simulink model "FinalTest_21_3"  (R2022b)
settings: Solver=FixedStepAuto  StartTime=0.0  StopTime=20  FixedStep=0.001  MaxStep=0.001  RelTol=1e-3
undefined symbols (not defined in the file): h, km, m, s, sigbuilder_block, smiData, X, Y, Z
libraries: sm_lib x105, aerolibconvert2 x14, nesl_utility x6, simulink_extras x4, vehdynlibsteering x1, autolibshared x1
(part 1 of 3)
settings Model: Creator=Lenovo  LastModifiedBy=Lenovo

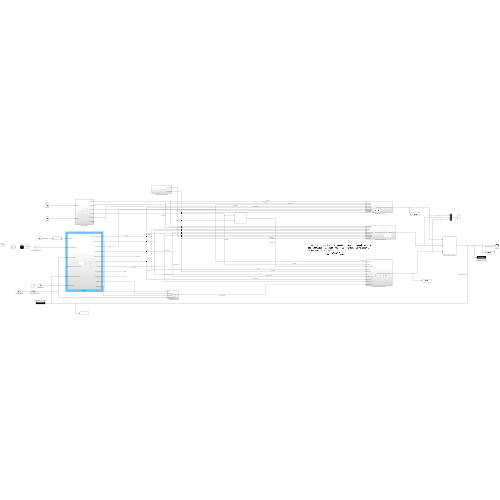
[thumbnail: Simulink's stored preview of the top-level diagram]
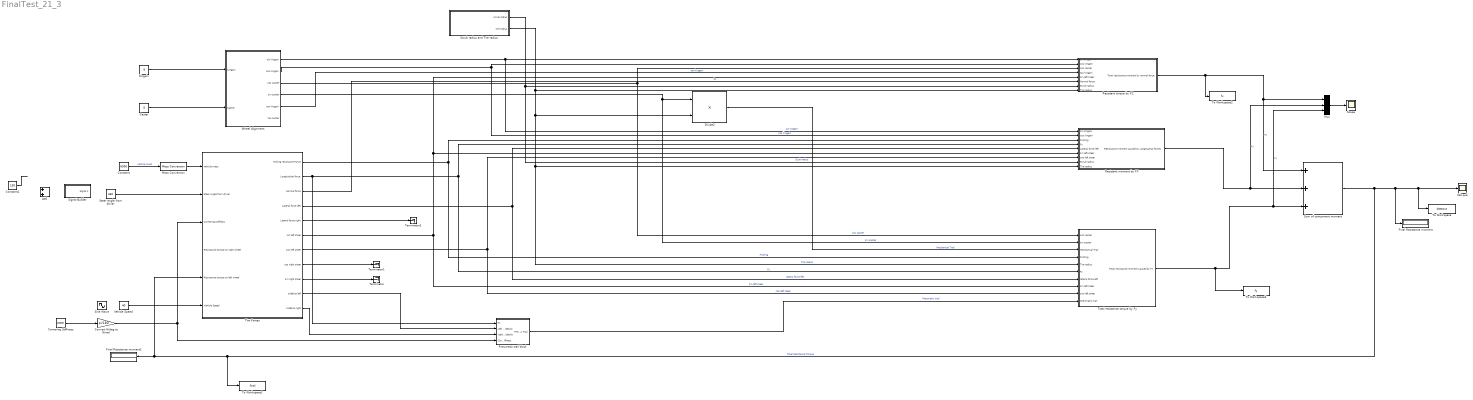
== system FinalTest_21_3 ==
  Add : Sum
  Caster : Constant  Value=5
  Constant : Constant  Value=6000
  Constant1 : Constant  Value=150
  Convert N/deg to N/rad : Gain  Gain=pi/180
  Cornering Stiffness : Constant  Value=20000
  Divide2 : Product  Inputs=**
  Final Resistance moment : Display
  Final Resistance moment1 : Display
  Kingpin : Constant  Value=9
  Kết quả : Scope
  Mass Conversion : aerolibconvert2/Mass Conversion  IU=kg  OU=kg
  Mux : Mux  Inputs=3
  Pneumatic trail block : Subsystem
  Resistant moment by FX : Subsystem
  Resistant torque by FZ : Subsystem
  Scope : Scope
  Scrub radius and Tire radius : Subsystem
  Signal Builder : Subsystem  Tag=STV Subsys  LoadFcn=sigbuilder_block('load');  StartFcn=sigbuilder_block('start');  StopFcn=sigbuilder_block('stop');  ClipboardFcn=sigbuilder_block('clipboard');  mask(Sigbuilder block){tuvar=[0:10]}
      mask help: Simulink:masks:SigbuilderBlock_MD
      mask init:
      | if ~strcmp(get_param(bdroot(gcbh),'SimulationStatus'),'stopped') tuvar = sigbuilder_block('maskInit'); end
      settings: CopyFcn=sigbuilder_block('copy');  DeleteFcn=sigbuilder_block('delete');  ModelCloseFcn=sigbuilder_block('modelClose');  PreSaveFcn=sigbuilder_block('preSave');  PauseFcn=sigbuilder_block('pause');  ContinueFcn=sigbuilder_block('continue');  NameChangeFcn=sigbuilder_block('namechange');  OpenFcn=sigbuilder_block('open',[437.6 199.2 550.4 400 ]);  CloseFcn=sigbuilder_block('close');
      mask Display: plot(0, 0, 100, 100,[2, 2, 32, 32, 2], [68, 8, 8, 68, 68],[32, 2], [38, 38], [32, 19, 2],[53, 60, 44], [32, 17, 17, 2],[16, 16, 31, 31]);txt = getActiveGroup(gcbh);text(2, 100, txt,'verticalAlignment', 'top');
  Sine Wave : Sin  Amplitude=60  SampleTime=0
  Steer angle from driver : Constant  Value=360
  Sum of component moment : Sum  Inputs=+++
  Terminator : Terminator
  Terminator1 : Terminator
  Terminator2 : Terminator
  Tire Forces : Subsystem
  To Workspace : ToWorkspace  VariableName=dataout  SaveFormat=Timeseries  SampleTime=-1
  To Workspace1 : ToWorkspace  VariableName=final  SaveFormat=Timeseries  SampleTime=-1
  To Workspace2 : ToWorkspace  VariableName=fx  SaveFormat=Timeseries  SampleTime=-1
  To Workspace3 : ToWorkspace  VariableName=fy  SaveFormat=Timeseries  SampleTime=-1
  Total resistance torque by Fy : Subsystem
  Vehicle Speed : Constant  Value=40
  Wheel Alignment : Subsystem
  wires:
  Constant/1 -> Mass Conversion/1  "vehicle mass"
  Tire Forces/3(Normal force) -> Resistant torque by FZ/6(Normal force)  "Fz"
  Tire Forces/5(Lateral force right) -> Terminator2/1
  Tire Forces/8(cos right steer) -> Terminator1/1
  Tire Forces/9(sin right steer) -> Terminator/1
  Kingpin/1 -> Wheel Alignment/1(Kingpin)
  Caster/1 -> Wheel Alignment/2(Caster)
  Wheel Alignment/4(sin caster) -> Total resistance torque by Fy/2(sin caster), Divide2/1  "sin caster"
  Wheel Alignment/1(sin kingpin) -> Resistant moment by FX/1(sin kingpin), Resistant torque by FZ/1(sin kingpin)  "sin kingpin"
  Wheel Alignment/2(cos kingpin) -> Resistant torque by FZ/2(cos kingpin), Resistant moment by FX/2(cos kingpin)  "cos kingpin"
  Wheel Alignment/3(cos caster) -> Total resistance torque by Fy/1(cos caster), Resistant torque by FZ/3(cos caster)  "cos caster"
  Wheel Alignment/5(tan kingpin) -> Resistant torque by FZ/4(tan kingpin)  "tan kingpin"
  Tire Forces/6(sin left steer) -> Total resistance torque by Fy/8(sin left steer), Resistant torque by FZ/5(sin left steer), Resistant moment by FX/6(sin left steer)  "sin left steer"
  Tire Forces/1(Rolling resistance Force) -> Resistant moment by FX/3(Frolling), Total resistance torque by Fy/4(Frolling)  "Frolling"
  Tire Forces/2(Longitudinal force) -> Pneumatic trail block/1(Fx), Total resistance torque by Fy/6(Fx), Resistant moment by FX/4(Fx)  "Fx"
  Tire Forces/4(Lateral force left) -> Total resistance torque by Fy/7(lateral force left), Resistant moment by FX/5(Lateral force left)  "lateral force left"
  Tire Forces/7(cos left steer) -> Total resistance torque by Fy/9(cos left steer), Resistant moment by FX/7(cos left steer)  "cos left steer"
  Cornering Stiffness/1 -> Convert N/deg to N/rad/1
  Tire Forces/10(sidelsip left) -> Pneumatic trail block/2(Left sideslip)
  Tire Forces/11(sideslip right) -> Pneumatic trail block/3(right sideslip)
  Scrub radius and Tire radius/2(tire radius) -> Total resistance torque by Fy/5(Tire radius), Resistant moment by FX/9(Tire radius), Divide2/2, Resistant torque by FZ/8(Tire radius)  "Tire radius"
  Scrub radius and Tire radius/1(scrub radius) -> Resistant moment by FX/8(Scrub radius), Resistant torque by FZ/7(Scrub radius)  "Scub radius"
  Divide2/1 -> Total resistance torque by Fy/3(Mechanical Trail)  "Mechanical Trail"
  Pneumatic trail block/1(Pneumatic Trail) -> Total resistance torque by Fy/10(pneumatic trail)  "Pneumatic trail"
  Resistant torque by FZ/1(Toral resistance moment by normal force) -> To Workspace2/1, Mux/1, Sum of component moment/1  "Fz"
  Total resistance torque by Fy/1(Total resistance moment caused by FY) -> To Workspace3/1, Mux/3, Sum of component moment/3  "Fy"
  Resistant moment by FX/1(Resistance moment caused by Longitudinal forces) -> Mux/2, Sum of component moment/2  "Fx"
  Mass Conversion/1 -> Tire Forces/1(vehicle mass)
  Sum of component moment/1 -> To Workspace1/1, Tire Forces/5("Resistance torque on left wheel "), Final Resistance moment1/1, To Workspace/1, Kết quả/1, Final Resistance moment/1  "Total Resstance Torque"
  Vehicle Speed/1 -> Tire Forces/6(Vehicle Speed)
  Convert N/deg to N/rad/1 -> Pneumatic trail block/4(Cornering Stiffness), Tire Forces/3(Cornering stiffness)
  Steer angle from driver/1 -> Tire Forces/2(Steer Angle from driver)
  Constant1/1 -> ?
  Mux/1 -> Scope/1

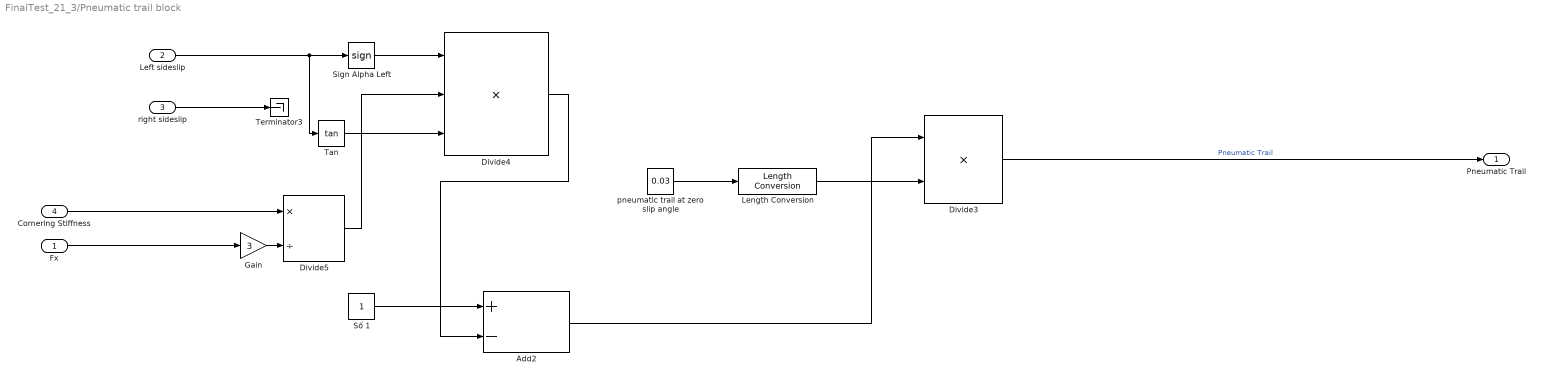
== system FinalTest_21_3/Pneumatic trail block ==
  Fx : Inport
  Left sideslip : Inport  Port=2
  right sideslip : Inport  Port=3
  Cornering Stiffness : Inport  Port=4
  Add2 : Sum  Inputs=+-
  Divide3 : Product  Inputs=**
  Divide4 : Product  Inputs=***
  Divide5 : Product  Inputs=*/
  Gain : Gain  Gain=3
  Length Conversion : aerolibconvert2/Length Conversion  IU=m  OU=m
  Sign Alpha Left : Signum
  Số 1 : Constant
  Tan : Trigonometry  Operator=tan
  Terminator3 : Terminator
  pneumatic trail at zero slip angle : Constant  Value=0.03
  Pneumatic Trail : Outport
  wires:
  Số 1/1 -> Add2/1
  Divide4/1 -> Add2/2
  Divide5/1 -> Divide4/2
  Tan/1 -> Divide4/3
  pneumatic trail at zero slip angle/1 -> Length Conversion/1
  Gain/1 -> Divide5/2
  Add2/1 -> Divide3/1
  Left sideslip/1 -> Tan/1, Sign Alpha Left/1
  Divide3/1 -> Pneumatic Trail/1  "Pneumatic Trail"
  right sideslip/1 -> Terminator3/1
  Fx/1 -> Gain/1
  Cornering Stiffness/1 -> Divide5/1
  Length Conversion/1 -> Divide3/2
  Sign Alpha Left/1 -> Divide4/1

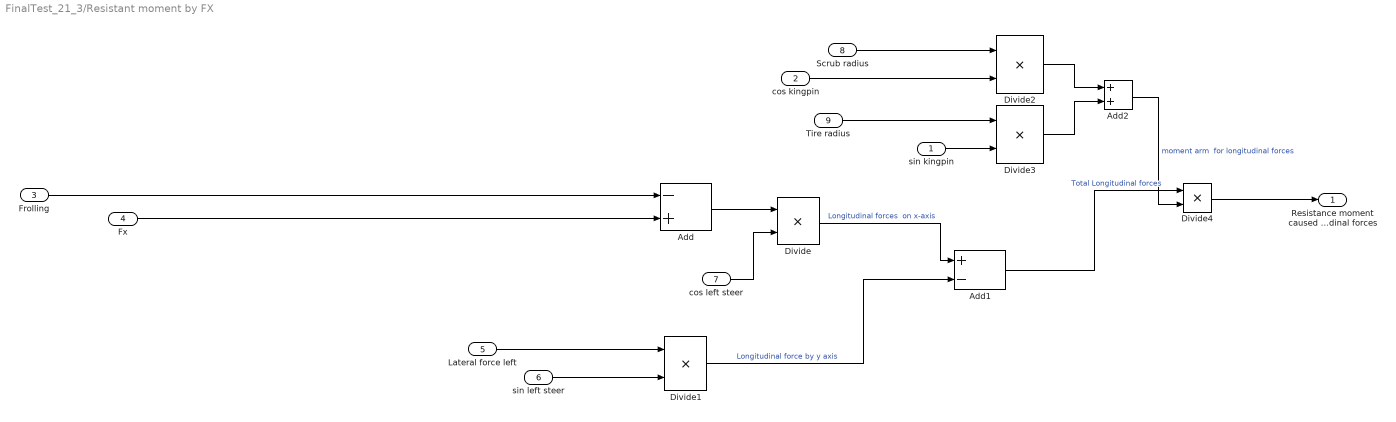
== system FinalTest_21_3/Resistant moment by FX ==
  sin kingpin : Inport
  cos kingpin : Inport  Port=2
  Frolling : Inport  Port=3
  Fx : Inport  Port=4
  Lateral force left : Inport  Port=5
  sin left steer : Inport  Port=6
  cos left steer : Inport  Port=7
  Scrub radius : Inport  Port=8
  Tire radius : Inport  Port=9
  Add : Sum  Inputs=-+
  Add1 : Sum  Inputs=+-
  Add2 : Sum
  Divide{,1..4} (5 alike) : Product  Inputs=**
  Resistance moment caused by Longitudinal forces : Outport
  wires:
  Scrub radius/1 -> Divide2/1
  Add1/1 -> Divide4/1  "Total Longitudinal forces"
  Divide/1 -> Add1/1  "Longitudinal forces  on x-axis"
  Divide1/1 -> Add1/2  "Longitudinal force by y axis"
  Lateral force left/1 -> Divide1/1
  Add/1 -> Divide/1
  Add2/1 -> Divide4/2  "moment arm  for longitudinal forces"
  Divide4/1 -> Resistance moment caused by Longitudinal forces/1
  Divide2/1 -> Add2/1
  Tire radius/1 -> Divide3/1
  Divide3/1 -> Add2/2
  cos kingpin/1 -> Divide2/2
  cos left steer/1 -> Divide/2
  sin left steer/1 -> Divide1/2
  Fx/1 -> Add/2
  Frolling/1 -> Add/1
  sin kingpin/1 -> Divide3/2

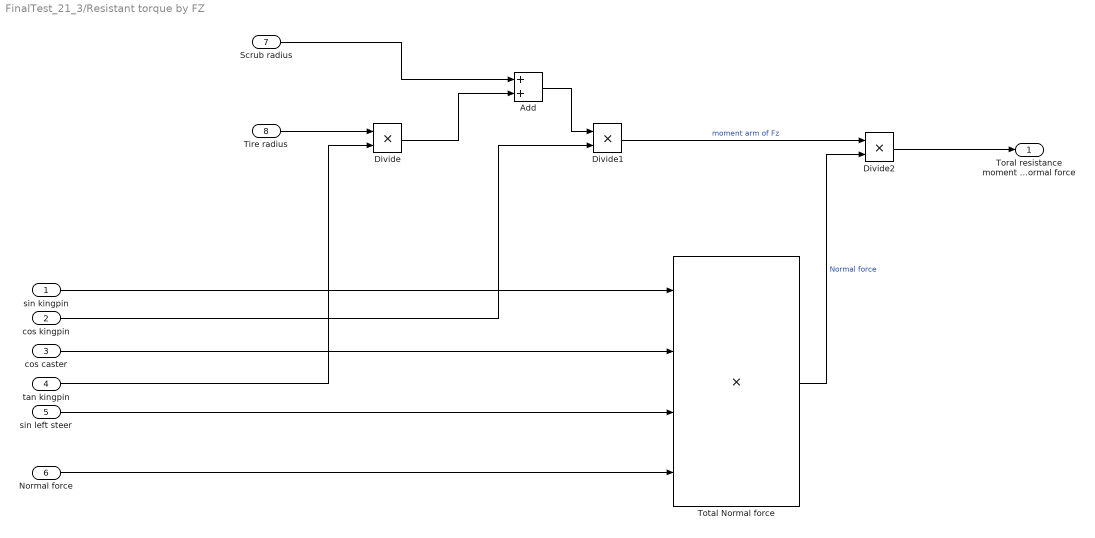
== system FinalTest_21_3/Resistant torque by FZ ==
  sin kingpin : Inport
  cos kingpin : Inport  Port=2
  cos caster : Inport  Port=3
  tan kingpin : Inport  Port=4
  sin left steer : Inport  Port=5
  Normal force : Inport  Port=6
  Scrub radius : Inport  Port=7
  Tire radius : Inport  Port=8
  Add : Sum
  Divide : Product  Inputs=**
  Divide1 : Product  Inputs=**
  Divide2 : Product  Inputs=**
  Total Normal force : Product  Inputs=****
  Toral resistance moment by normal force : Outport
  wires:
  Tire radius/1 -> Divide/1
  cos kingpin/1 -> Divide1/2
  sin kingpin/1 -> Total Normal force/1
  Scrub radius/1 -> Add/1
  Total Normal force/1 -> Divide2/2  "Normal force"
  Divide1/1 -> Divide2/1  "moment arm of Fz"
  Divide/1 -> Add/2
  Add/1 -> Divide1/1
  cos caster/1 -> Total Normal force/2
  sin left steer/1 -> Total Normal force/3
  tan kingpin/1 -> Divide/2
  Divide2/1 -> Toral resistance moment by normal force/1
  Normal force/1 -> Total Normal force/4

== system FinalTest_21_3/Scrub radius and Tire radius ==
  Length Conversion : aerolibconvert2/Length Conversion  IU=m  OU=m
  Length Conversion1 : aerolibconvert2/Length Conversion  IU=m  OU=m
  Scrub radius : Constant  Value=0.01
  Tire radius : Constant  Value=0.187
  scrub radius : Outport
  tire radius : Outport  Port=2
  wires:
  Tire radius/1 -> Length Conversion1/1  "tire radius"
  Scrub radius/1 -> Length Conversion/1  "scrub radius"
  Length Conversion/1 -> scrub radius/1
  Length Conversion1/1 -> tire radius/1

== system FinalTest_21_3/Signal Builder ==
  Demux : Demux  Tag=STV Demux  Outputs=1
      settings: DisplayOption=none
  FromWs : FromWorkspace  Tag=STV FromWs  VariableName=tuvar
      SigBuilderData=|
      | common.afterFinalStr = 'Extrapolate'
      | common.sampleTime = 0
      | dataSet.timeRange = [0 10]
      | dataSet.name = 'Group 1'
      | sbobj.Groups.Name = 'Group 1'
      | sbobj.Groups.Signals.Name = 'Signal 1'
      | sbobj.Groups.Signals.XData = [0 1.98 1.98 4.04 4.04 10]
      | sbobj.Groups.Signals.YData = [90 90 180 180 220 220]
  Signal 1 : Outport  Tag=STV Outport
  wires:
  Demux/1 -> Signal 1/1
  FromWs/1 -> Demux/1

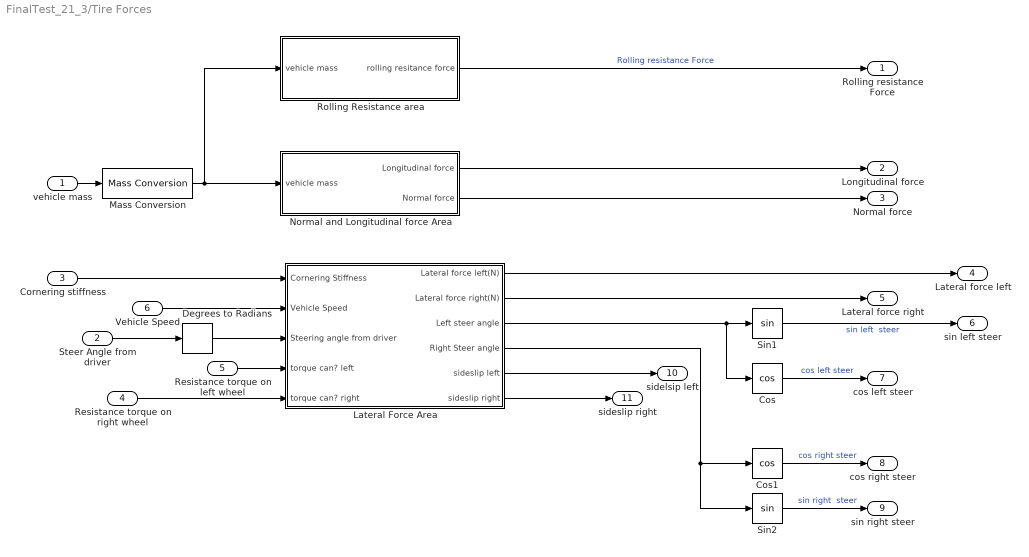
== system FinalTest_21_3/Tire Forces ==
  vehicle mass : Inport
  Steer Angle from driver : Inport  Port=2
  Cornering stiffness : Inport  Port=3
  "Resistance torque on right wheel " : Inport  Port=4
  "Resistance torque on left wheel " : Inport  Port=5
  Vehicle Speed : Inport  Port=6
  Cos : Trigonometry  Operator=cos
  Cos1 : Trigonometry  Operator=cos
  Degrees to Radians : simulink_extras/Transformations/Degrees to Radians
  Lateral Force Area : Subsystem
  Mass Conversion : aerolibconvert2/Mass Conversion  IU=kg  OU=kg
  Normal and Longitudinal force Area : Subsystem
  Rolling Resistance area : Subsystem
  Sin1 : Trigonometry
  Sin2 : Trigonometry
  Rolling resistance Force : Outport
  Longitudinal force : Outport  Port=2
  Normal force : Outport  Port=3
  Lateral force left : Outport  Port=4
  Lateral force right : Outport  Port=5
  sin left steer : Outport  Port=6
  cos left steer : Outport  Port=7
  cos right steer : Outport  Port=8
  sin right steer : Outport  Port=9
  sidelsip left : Outport  Port=10
  sideslip right : Outport  Port=11
  wires:
  Degrees to Radians/1 -> Lateral Force Area/3(Steering angle from driver)
  Lateral Force Area/4(Right Steer angle) -> Sin2/1, Cos1/1
  vehicle mass/1 -> Mass Conversion/1
  Sin2/1 -> sin right steer/1  "sin right  steer"
  Cos1/1 -> cos right steer/1  "cos right steer"
  Lateral Force Area/3(Left steer angle) -> Cos/1, Sin1/1
  Normal and Longitudinal force Area/1(Longitudinal force) -> Longitudinal force/1
  Normal and Longitudinal force Area/2(Normal force) -> Normal force/1
  Sin1/1 -> sin left steer/1  "sin left  steer"
  Rolling Resistance area/1(rolling resitance force) -> Rolling resistance Force/1  "Rolling resistance Force"
  Steer Angle from driver/1 -> Degrees to Radians/1
  Cos/1 -> cos left steer/1  "cos left steer"
  Lateral Force Area/2("Lateral force right(N)  ") -> Lateral force right/1
  Lateral Force Area/1(Lateral force left(N)) -> Lateral force left/1
  Lateral Force Area/5(sideslip left) -> sidelsip left/1
  Lateral Force Area/6("sideslip right ") -> sideslip right/1
  Cornering stiffness/1 -> Lateral Force Area/1("Cornering Stiffness ")
  Mass Conversion/1 -> Rolling Resistance area/1(vehicle mass), Normal and Longitudinal force Area/1(vehicle mass)
  Vehicle Speed/1 -> Lateral Force Area/2(Vehicle Speed)
  "Resistance torque on left wheel "/1 -> Lateral Force Area/4(torque can? left)
  "Resistance torque on right wheel "/1 -> Lateral Force Area/5(torque can? right)

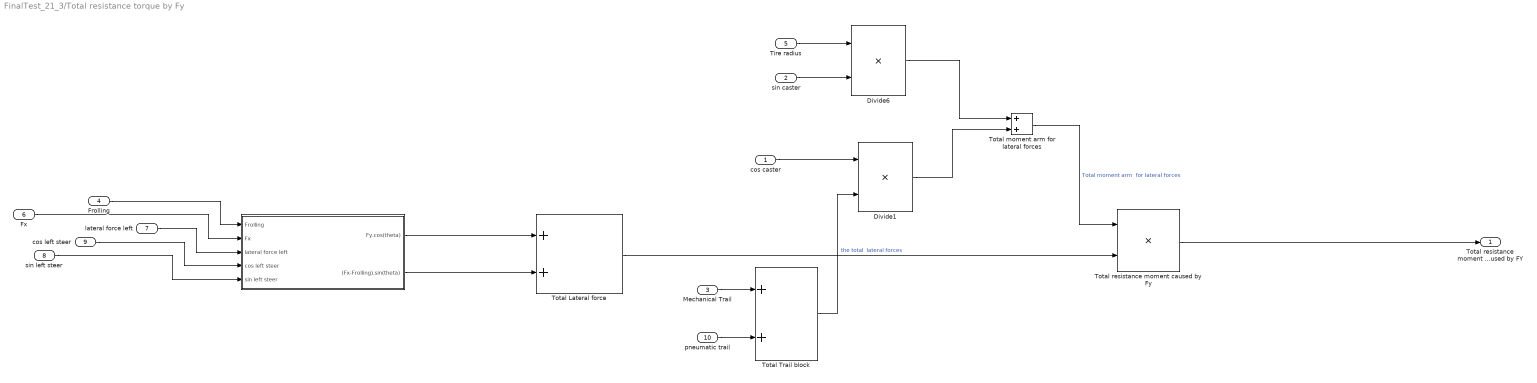
== system FinalTest_21_3/Total resistance torque by Fy ==
  cos caster : Inport
  sin caster : Inport  Port=2
  Mechanical Trail : Inport  Port=3
  Frolling : Inport  Port=4
  Tire radius : Inport  Port=5
  Fx : Inport  Port=6
  lateral force left : Inport  Port=7
  sin left steer : Inport  Port=8
  cos left steer : Inport  Port=9
  pneumatic trail : Inport  Port=10
  " " : Subsystem
  Divide1 : Product  Inputs=**
  Divide6 : Product  Inputs=**
  Total Lateral force : Sum
  Total Trail block : Sum
  Total moment arm for lateral forces : Sum
  Total resistance moment caused by Fy : Product  Inputs=**
  Total resistance moment caused by FY : Outport
  wires:
  cos caster/1 -> Divide1/1
  Divide6/1 -> Total moment arm for lateral forces/1
  Total moment arm for lateral forces/1 -> Total resistance moment caused by Fy/1  "Total moment arm  for lateral forces"
  Total Lateral force/1 -> Total resistance moment caused by Fy/2  "the total  lateral forces"
  Divide1/1 -> Total moment arm for lateral forces/2
  " "/1(Fy.cos(theta)) -> Total Lateral force/1
  Total Trail block/1 -> Divide1/2
  " "/2((Fx-Frolling).sin(theta)) -> Total Lateral force/2
  Total resistance moment caused by Fy/1 -> Total resistance moment caused by FY/1
  pneumatic trail/1 -> Total Trail block/2
  Tire radius/1 -> Divide6/1
  sin caster/1 -> Divide6/2
  cos left steer/1 -> " "/4(cos left steer)
  Frolling/1 -> " "/1(Frolling)
  lateral force left/1 -> " "/3(lateral force left)
  sin left steer/1 -> " "/5(sin left steer)
  Fx/1 -> " "/2(Fx)
  Mechanical Trail/1 -> Total Trail block/1

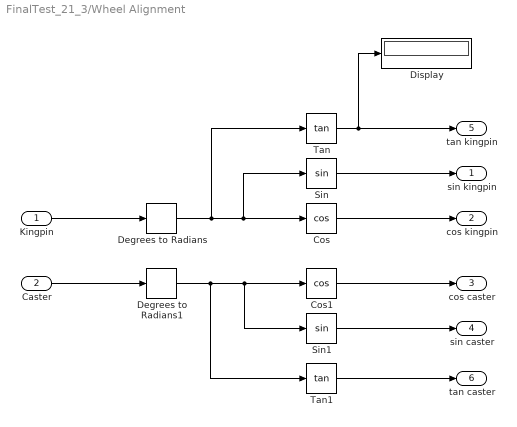
== system FinalTest_21_3/Wheel Alignment ==
  Kingpin : Inport
  Caster : Inport  Port=2
  Cos : Trigonometry  Operator=cos
  Cos1 : Trigonometry  Operator=cos
  Degrees to Radians : simulink_extras/Transformations/Degrees to Radians
  Degrees to Radians1 : simulink_extras/Transformations/Degrees to Radians
  Display : Display
  Sin : Trigonometry
  Sin1 : Trigonometry
  Tan : Trigonometry  Operator=tan
  Tan1 : Trigonometry  Operator=tan
  sin kingpin : Outport
  cos kingpin : Outport  Port=2
  cos caster : Outport  Port=3
  sin caster : Outport  Port=4
  tan kingpin : Outport  Port=5
  tan caster : Outport  Port=6
  wires:
  Sin1/1 -> sin caster/1
  Degrees to Radians1/1 -> Tan1/1, Sin1/1, Cos1/1
  Sin/1 -> sin kingpin/1
  Caster/1 -> Degrees to Radians1/1
  Cos1/1 -> cos caster/1
  Cos/1 -> cos kingpin/1
  Degrees to Radians/1 -> Tan/1, Sin/1, Cos/1
  Kingpin/1 -> Degrees to Radians/1
  Tan/1 -> Display/1, tan kingpin/1
  Tan1/1 -> tan caster/1

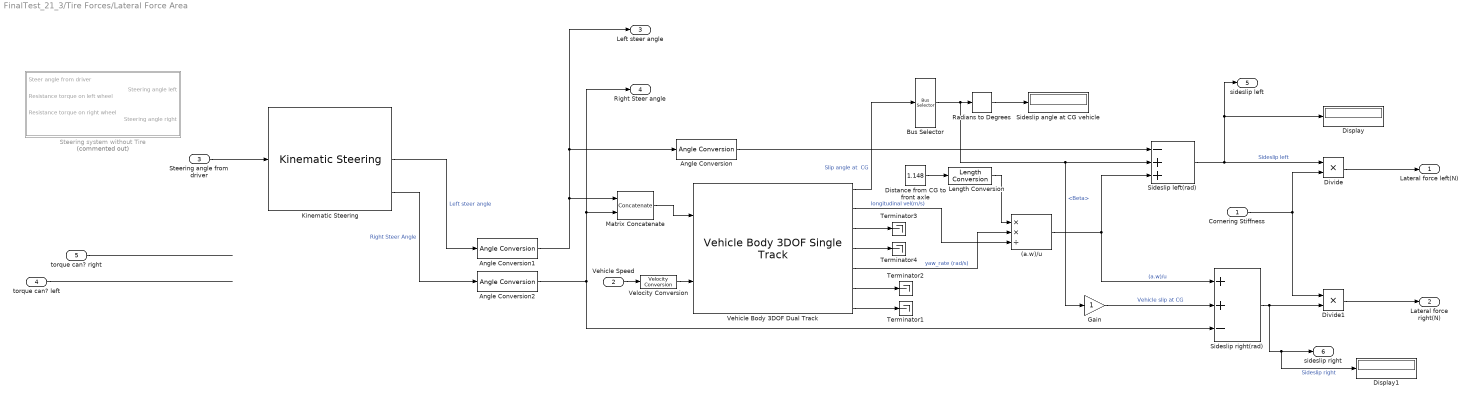
== system FinalTest_21_3/Tire Forces/Lateral Force Area ==
  "Cornering Stiffness " : Inport
  Vehicle Speed : Inport  Port=2
  Steering angle from driver : Inport  Port=3
  torque can? left : Inport  Port=4
  torque can? right : Inport  Port=5
  (a.w)/u : Product  Inputs=**/
  Angle Conversion : aerolibconvert2/Angle Conversion  IU=rad  OU=rad
  Angle Conversion1 : aerolibconvert2/Angle Conversion  IU=rad  OU=rad
  Angle Conversion2 : aerolibconvert2/Angle Conversion  IU=rad  OU=rad
  Bus Selector : BusSelector  OutputSignals=BdyFrm.Cg.Ang.Beta
  Display : Display
  Display1 : Display
  Distance from CG to front axle : Constant  Value=1.148
  Divide : Product  Inputs=**
  Divide1 : Product  Inputs=**
  Gain : Gain
  Kinematic Steering : vehdynlibsteering/Kinematic Steering  StrgType=Rack and pinion  StrgRatioType=Constant  Loc=Front  NrmlFctr=0.01  TrckWdth=1.4  WhlBase=1.524  Db=0  StrgRng=4*pi  StrgAngBpts="[-6.2832   -5.0265   -3.7699   -2.5133   -1.2566         0    1.2566    2.5133    3.7699    5.0265    6.2832]"  StrgRatioTbl=|  StrgRatio=100  PctAckIn=off  PctAck=100  PctAckTbl=ones(1,11)*100  StrgArmLngth=0.2  RckCsLngth=0.6  TieRodLngth=0.248  D=0.2  PnnRadius=0.03  PnnRadiusTbl="[0.0055    0.0055    0.0056    0.0057    0.0058    0.0057    0.0057    0.0057    0.0056    0.0055    0.0055]"  RodLngth=0.1  ParaArmLngth=0.9  aMode=2
      | [13.5000   13.3750   13.2500   13.1250   13.0000   13.0000   13.0000   13.1250   13.2500   13.3750   13.5000
      | ]
  Length Conversion : aerolibconvert2/Length Conversion  IU=m  OU=m
  Matrix Concatenate : Concatenate  ConcatenateDimension=2
  Radians to Degrees : simulink_extras/Transformations/Radians to Degrees
  Sideslip angle at CG vehicle : Display
  "Sideslip left(rad) " : Sum  Inputs=-++
  Sideslip right(rad) : Sum  Inputs=++-
  Steering system without Tire : Subsystem  Commented=on
  Terminator{1..4} (4 alike) : Terminator
  Vehicle Body 3DOF Dual Track : autolibshared/Vehicle Body 3DOF Single Track  trackMode=Dual  inputMode=External longitudinal velocity  frontSteerMode=on  rearSteerMode=off  windMode=off  muMode=off  extFMode=off  extMMode=off  htchFMode=off  htchMMode=off  extXo=off  extpsio=off  extxdoto=off  extro=off  extYo=off  extTamb=off  extydoto=off  aMode=2  NF=2  NR=2  m=4000  a=1.148  b=1.402  h=0.2  dh=1  hh=0.2  X_o=0  xdot_o=0  CalphaMode=off  sigmaMode=on  d=0  hl=0  w=[1.4,1.4]  Cy_f=350  Cy_r=500  sigma_f=.01  sigma_r=.1  alpha_f_brk=[-.1 .1]  Cy_f_data=[-9e3 9e3]  alpha_r_brk=[-.1 .1]  Cy_r_data=[-9e3 9e3]  Y_o=0  ydot_o=0  Izz=3600  psi_o=0  r_o=0  Af=2  Cd=.3  Cl=.1  Cpm=.1  beta_w=[0 0.01:0.01:0.3]  Cs=[0:0.03:0.9]  Cym=[0 1e-6:0.01:0.3]  Pabs=101325  Tair=273  g=9.81  mu=1  xdot_tol=.001  Fznom=13467  Fxtire_sat=7e4  Fytire_sat=7e4  longOff=0  latOff=0  vertOff=0  wrapAng=off
      settings: LibrarySourceBlock=vehdynlibeom/Vehicle Body 3DOF Dual Track
  Velocity Conversion : aerolibconvert2/Velocity Conversion  IU=km/h  OU=m/s
  Lateral force left(N) : Outport
  "Lateral force right(N)  " : Outport  Port=2
  Left steer angle : Outport  Port=3
  Right Steer angle : Outport  Port=4
  sideslip left : Outport  Port=5
  "sideslip right " : Outport  Port=6
  wires:
  Radians to Degrees/1 -> Sideslip angle at CG vehicle/1
  Sideslip right(rad)/1 -> Display1/1, "sideslip right "/1, Divide1/2  "Sideslip right"
  Vehicle Body 3DOF Dual Track/4 -> Terminator4/1
  Vehicle Body 3DOF Dual Track/6 -> Terminator2/1
  Kinematic Steering/2 -> Angle Conversion1/1  "Left steer angle"
  (a.w)/u/1 -> Sideslip right(rad)/1, "Sideslip left(rad) "/3  "(a.w)/u"
  Gain/1 -> Sideslip right(rad)/2  "Vehicle slip at CG"
  Distance from CG to front axle/1 -> Length Conversion/1
  Matrix Concatenate/1 -> Vehicle Body 3DOF Dual Track/1
  Bus Selector/1 -> Gain/1, "Sideslip left(rad) "/2, Radians to Degrees/1  "<Beta>"
  "Cornering Stiffness "/1 -> Divide1/1, Divide/2
  Vehicle Speed/1 -> Velocity Conversion/1
  Vehicle Body 3DOF Dual Track/2 -> (a.w)/u/3  "longitudinal vel(m/s)"
  Vehicle Body 3DOF Dual Track/1 -> Bus Selector/1  "Slip angle at  CG"
  Kinematic Steering/3 -> Angle Conversion2/1  "Right Steer Angle"
  Divide1/1 -> "Lateral force right(N)  "/1
  "Sideslip left(rad) "/1 -> sideslip left/1, Display/1, Divide/1  "Sideslip left"
  Vehicle Body 3DOF Dual Track/5 -> (a.w)/u/2  "yaw_rate (rad/s)"
  Vehicle Body 3DOF Dual Track/7 -> Terminator1/1
  Divide/1 -> Lateral force left(N)/1
  Velocity Conversion/1 -> Vehicle Body 3DOF Dual Track/2
  Length Conversion/1 -> (a.w)/u/1
  Angle Conversion/1 -> "Sideslip left(rad) "/1
  Angle Conversion1/1 -> Left steer angle/1, Angle Conversion/1, Matrix Concatenate/1
  Angle Conversion2/1 -> Right Steer angle/1, Matrix Concatenate/2, Sideslip right(rad)/3
  Steering angle from driver/1 -> Kinematic Steering/1
  torque can? left/1 -> ?
  torque can? right/1 -> ?
  Vehicle Body 3DOF Dual Track/3 -> Terminator3/1

== system FinalTest_21_3/Tire Forces/Normal and Longitudinal force Area ==
  vehicle mass : Inport
  Longitudinal Friction Coefficient : Gain  Gain=0.35
  Normal Force : Subsystem
  Longitudinal force : Outport
  Normal force : Outport  Port=2
  wires:
  Normal Force/1(Fz) -> Normal force/1, Longitudinal Friction Coefficient/1
  Longitudinal Friction Coefficient/1 -> Longitudinal force/1
  vehicle mass/1 -> Normal Force/1(In1)

== system FinalTest_21_3/Tire Forces/Rolling Resistance area ==
  vehicle mass : Inport
  Acceleration Conversion : aerolibconvert2/Acceleration Conversion  IU=m/s^2  OU=m/s^2
  Divide : Product  Inputs=***
  Gravity : Constant  Value=9.81
  Rolling resitance coefficient : Constant  Value=0.011
  rolling resitance force : Outport
  wires:
  Rolling resitance coefficient/1 -> Divide/3
  Gravity/1 -> Acceleration Conversion/1
  Divide/1 -> rolling resitance force/1  "rolling resitance force"
  vehicle mass/1 -> Divide/1
  Acceleration Conversion/1 -> Divide/2

== system FinalTest_21_3/Total resistance torque by Fy/  ==
  Frolling : Inport
  Fx : Inport  Port=2
  lateral force left : Inport  Port=3
  cos left steer : Inport  Port=4
  sin left steer : Inport  Port=5
  Add : Sum  Inputs=+-
  Divide : Product  Inputs=**
  Divide1 : Product  Inputs=**
  Fy.cos(theta) : Outport
  (Fx-Frolling).sin(theta) : Outport  Port=2
  wires:
  Divide1/1 -> (Fx-Frolling).sin(theta)/1  "(Fx-Frolling).sin(theta)"
  Add/1 -> Divide1/1
  Frolling/1 -> Add/2
  lateral force left/1 -> Divide/1
  cos left steer/1 -> Divide/2
  sin left steer/1 -> Divide1/2
  Fx/1 -> Add/1
  Divide/1 -> Fy.cos(theta)/1  "Fy.cos(theta)"

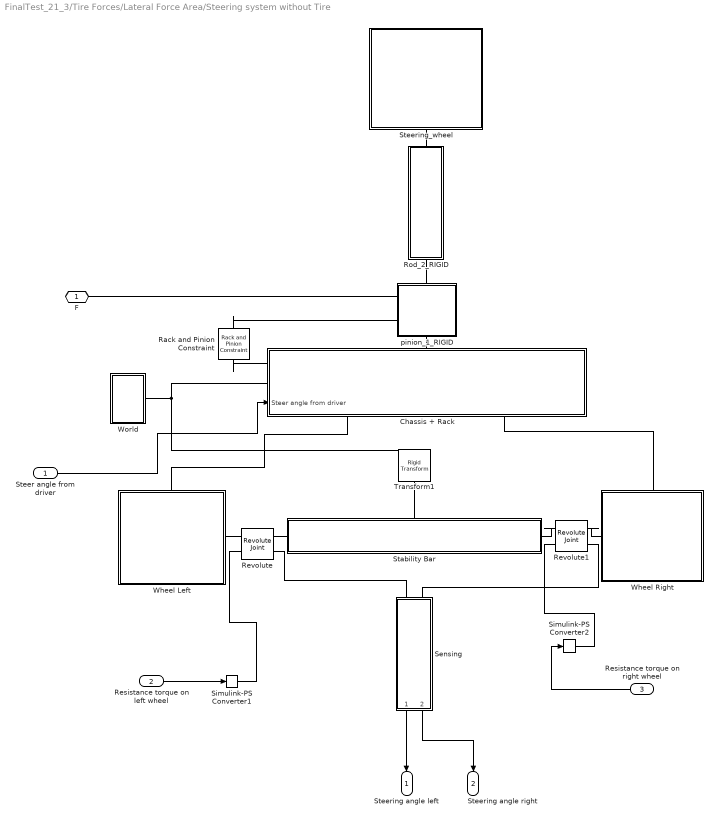
== system FinalTest_21_3/Tire Forces/Lateral Force Area/Steering system without Tire ==
  Steer angle from driver : Inport
  "Resistance torque on left wheel " : Inport  Port=2
  "Resistance torque on right wheel " : Inport  Port=3
  Chassis + Rack : Subsystem
      settings: PortSchema="{\"entries\":[{\"content\":{\"sides\":[{\"content\":{\"connectorIds\":[\"LConn1\",\"LConn2\",\"In1\"]},\"type\":\"ConnectorPlacement.EquallySpacedRectSide\",\"uuid\":\"238826d0-ecaf-49b3-85a0-aed5fbc0c007\"},{\"content\":{\"connectorIds\":[],\"side\":\"RIGHT\"},\"type\":\"ConnectorPlacement.EquallySpacedRectSide\",\"uuid\":\"b2c6ab3d-7118-49e7-a9c5-d2df9074f914\"},{\"content\":{\"connectorIds\":[\"LConn3\"],\"side\":\"TOP\"},\"type\":\"ConnectorPlacement.EquallySpacedRectSide\",\"uuid\":\"7d2cd5c8-d305-43dc-8ebb-f8d67bbd0110\"},{\"content\":{\"connectorIds\":[\"RConn1\",\"RConn2\"],\"side\":\"BOTTOM\"},\"type\":\"ConnectorPlacement.EquallySpacedRectSide\",\"uuid\":\"2aef2c72-a8ff-4d58-b95f-1e6acc753e3a\"}]},\"type\":\"ConnectorPlacement.EquallySpacedConnector\",\"uuid\":\"1f5b54f8-4c78-4fbe-ac16-0d340b3ede3d\"}],\"packageUris\":[\"http://schema.mathworks.com/mf0/Connector/R2020b\"],\"version\":\"1.0\"}"
      mask Display: image('E:\Hoc\do an\(final) download\test14\image\Chassis+rack.png'); % Use "Edit Image" on toolstrip to change.
  Rack and Pinion Constraint : sm_lib/Gears and Couplings/Gears/Rack and Pinion Constraint  PinionRadius=30  PinionRadiusUnits=mm
  Revolute : sm_lib/Joints/Revolute Joint  JointMode=Normal  SenseConstraintForce=off  SenseConstraintForceX=off  SenseConstraintForceY=off  SenseConstraintForceZ=off  SenseConstraintTorque=off  SenseConstraintTorqueX=off  SenseConstraintTorqueY=off  SenseConstraintTorqueZ=off  SenseTotalForce=off  SenseTotalForceX=off  SenseTotalForceY=off  SenseTotalForceZ=off  SenseTotalTorque=off  SenseTotalTorqueX=off  SenseTotalTorqueY=off  SenseTotalTorqueZ=off  CompositeWrenchDir=FollowerOnBase  CompositeWrenchFrame=BaseFrame  EquilibriumPosition=0  EquilibriumPositionUnits=deg  SpringStiffness=0  SpringStiffnessUnits=N*m/deg  DampingCoefficient=1.5  DampingCoefficientUnits=N*m/(deg/s)  TorqueActuationMode=InputTorque  MotionActuationMode=ComputedMotion  SensePosition=on  SenseVelocity=off  SenseAcceleration=off  SenseTorqueForce=off  SenseLowerLimitTorqueForce=off  SenseUpperLimitTorqueForce=off  LowerLimitSpecify=off  LowerLimitBound=-2  LowerLimitBoundUnits=rad  LowerLimitStiffness=1e4  LowerLimitStiffnessUnits=N*m/deg  LowerLimitDamping=10  LowerLimitDampingUnits=N*m/(deg/s)  LowerLimitTransitionRegionWidth=0.1  LowerLimitTransitionRegionWidthUnits=deg  UpperLimitSpecify=off  UpperLimitBound=-1.14  UpperLimitBoundUnits=rad  UpperLimitStiffness=1e4  UpperLimitStiffnessUnits=N*m/deg  UpperLimitDamping=10  UpperLimitDampingUnits=N*m/(deg/s)  UpperLimitTransitionRegionWidth=0.1  UpperLimitTransitionRegionWidthUnits=deg  PositionTargetSpecify=on  PositionTargetPriority=Low  PositionTargetValue=smiData.RevoluteJoint(1).Rz.Pos  PositionTargetValueUnits=deg  VelocityTargetSpecify=off  VelocityTargetPriority=High  VelocityTargetValue=0  VelocityTargetValueUnits=deg/s
  Revolute1 : sm_lib/Joints/Revolute Joint  JointMode=Normal  SenseConstraintForce=off  SenseConstraintForceX=off  SenseConstraintForceY=off  SenseConstraintForceZ=off  SenseConstraintTorque=off  SenseConstraintTorqueX=off  SenseConstraintTorqueY=off  SenseConstraintTorqueZ=off  SenseTotalForce=off  SenseTotalForceX=off  SenseTotalForceY=off  SenseTotalForceZ=off  SenseTotalTorque=off  SenseTotalTorqueX=off  SenseTotalTorqueY=off  SenseTotalTorqueZ=off  CompositeWrenchDir=FollowerOnBase  CompositeWrenchFrame=BaseFrame  EquilibriumPosition=0  EquilibriumPositionUnits=deg  SpringStiffness=0  SpringStiffnessUnits=N*m/deg  DampingCoefficient=1.5  DampingCoefficientUnits=N*m/(deg/s)  TorqueActuationMode=InputTorque  MotionActuationMode=ComputedMotion  SensePosition=on  SenseVelocity=off  SenseAcceleration=off  SenseTorqueForce=off  SenseLowerLimitTorqueForce=off  SenseUpperLimitTorqueForce=off  LowerLimitSpecify=off  LowerLimitBound=-2  LowerLimitBoundUnits=rad  LowerLimitStiffness=1e4  LowerLimitStiffnessUnits=N*m/deg  LowerLimitDamping=10  LowerLimitDampingUnits=N*m/(deg/s)  LowerLimitTransitionRegionWidth=0.1  LowerLimitTransitionRegionWidthUnits=deg  UpperLimitSpecify=off  UpperLimitBound=-1.14  UpperLimitBoundUnits=rad  UpperLimitStiffness=1e4  UpperLimitStiffnessUnits=N*m/deg  UpperLimitDamping=10  UpperLimitDampingUnits=N*m/(deg/s)  UpperLimitTransitionRegionWidth=0.1  UpperLimitTransitionRegionWidthUnits=deg  PositionTargetSpecify=on  PositionTargetPriority=Low  PositionTargetValue=smiData.RevoluteJoint(2).Rz.Pos  PositionTargetValueUnits=deg  VelocityTargetSpecify=off  VelocityTargetPriority=High  VelocityTargetValue=0  VelocityTargetValueUnits=deg/s
  Rod_2_RIGID : Subsystem
      mask Display: image('E:\Hoc\do an\(final) download\test14\image\rod.png'); % Use "Edit Image" on toolstrip to change.
  "Sensing " : Subsystem
  Simulink-PS Converter1 : nesl_utility/Simulink-PS Converter  PhysicalDomain=network_engine_domain  SubClassName=ps_input  LeftPortType=input  RightPortType=output  PseudoPeriodic=off  Frequencies=[]  NoiseDistribution=none  NoiseParameters=[]  Unit=1  AffineConversion=off  FilteringAndDerivatives=provide  SimscapeFilterOrder=1  InputFilterTimeConstant=0.001  UdotUserProvided=0
  Simulink-PS Converter2 : nesl_utility/Simulink-PS Converter  PhysicalDomain=network_engine_domain  SubClassName=ps_input  LeftPortType=input  RightPortType=output  PseudoPeriodic=off  Frequencies=[]  NoiseDistribution=none  NoiseParameters=[]  Unit=1  AffineConversion=off  FilteringAndDerivatives=provide  SimscapeFilterOrder=1  InputFilterTimeConstant=0.001  UdotUserProvided=0
  Stability Bar : Subsystem
      settings: PortSchema="{\"entries\":[{\"content\":{\"sides\":[{\"content\":{\"connectorIds\":[\"LConn1\"]},\"type\":\"ConnectorPlacement.EquallySpacedRectSide\",\"uuid\":\"d47e2ccc-0711-4778-98f2-db3de543764b\"},{\"content\":{\"connectorIds\":[\"RConn1\"],\"side\":\"RIGHT\"},\"type\":\"ConnectorPlacement.EquallySpacedRectSide\",\"uuid\":\"6519cf91-ea6a-455a-8d22-5a1b5115bdd1\"},{\"content\":{\"connectorIds\":[\"LConn2\"],\"side\":\"TOP\"},\"type\":\"ConnectorPlacement.EquallySpacedRectSide\",\"uuid\":\"0f517cd1-9621-44ed-8d3d-d2d0bec2d80f\"}]},\"type\":\"ConnectorPlacement.EquallySpacedConnector\",\"uuid\":\"c248e281-f8e7-4e5b-ada2-47cc777e60c1\"}],\"packageUris\":[\"http://schema.mathworks.com/mf0/Connector/R2020b\"],\"version\":\"1.0\"}"
      mask Display: image('E:\Hoc\do an\(final) download\test14\image\stability bar.png'); % Use "Edit Image" on toolstrip to change.
  Steering_wheel : Subsystem
      mask Display: image('steering wheel.png'); % Use "Edit Image" on toolstrip to change.
  Transform1 : sm_lib/Frames and Transforms/Rigid Transform  TranslationMethod=Cartesian  TranslationStandardOffset=0  TranslationLengthUnit=mm  TranslationStandardAxis=+Z  TranslationCartesianOffset=smiData.RigidTransform(48).translation  TranslationROffset=0  TranslationROffsetUnits=m  TranslationZOffset=0  TranslationZOffsetUnits=m  TranslationThetaOffset=0  TranslationThetaOffsetUnits=deg  RotationMethod=ArbitraryAxis  RotationAngleUnits=rad  RotationStandardAxis=+Z  RotationAngle=smiData.RigidTransform(48).angle  RotationArbitraryAxis=smiData.RigidTransform(48).axis  FollAlignAxisA=+X  BaseAlignAxisA=+Y  FollAlignAxisB=+Y  BaseAlignAxisB=+Z  RotationSequenceAxes=FollowerAxes  RotationSequence=XYX  RotationSequenceAngles=[0 0 0]  RotationSequenceAnglesUnits=deg  RotationMatrix=[1 0 0; 0 1 0; 0 0 1]  Quaternion=[1 0 0 0]
  Wheel Left : Subsystem
      settings: PortSchema="{\"entries\":[{\"content\":{\"sides\":[{\"content\":{\"connectorIds\":[]},\"type\":\"ConnectorPlacement.EquallySpacedRectSide\",\"uuid\":\"8ca227ee-ead8-4d63-82a5-5856c0dfeded\"},{\"content\":{\"connectorIds\":[\"RConn1\"],\"side\":\"RIGHT\"},\"type\":\"ConnectorPlacement.EquallySpacedRectSide\",\"uuid\":\"8b239547-5df1-40f8-9337-2447adaec5b2\"},{\"content\":{\"connectorIds\":[\"LConn1\"],\"side\":\"TOP\"},\"type\":\"ConnectorPlacement.EquallySpacedRectSide\",\"uuid\":\"f7fdfa0e-4b43-4c5b-9845-cbdb5b136f6f\"}]},\"type\":\"ConnectorPlacement.EquallySpacedConnector\",\"uuid\":\"60e52eb2-18eb-41a9-88d9-70caa688cc15\"}],\"packageUris\":[\"http://schema.mathworks.com/mf0/Connector/R2020b\"],\"version\":\"1.0\"}"
      mask Display: image('E:\Hoc\do an\(final) download\test14\image\wheel.png'); % Use "Edit Image" on toolstrip to change.
  Wheel Right : Subsystem
      settings: PortSchema="{\"entries\":[{\"content\":{\"sides\":[{\"content\":{\"connectorIds\":[\"LConn1\"]},\"type\":\"ConnectorPlacement.EquallySpacedRectSide\",\"uuid\":\"8ca227ee-ead8-4d63-82a5-5856c0dfeded\"},{\"content\":{\"connectorIds\":[],\"side\":\"RIGHT\"},\"type\":\"ConnectorPlacement.EquallySpacedRectSide\",\"uuid\":\"8b239547-5df1-40f8-9337-2447adaec5b2\"},{\"content\":{\"connectorIds\":[\"LConn2\"],\"side\":\"TOP\"},\"type\":\"ConnectorPlacement.EquallySpacedRectSide\",\"uuid\":\"f7fdfa0e-4b43-4c5b-9845-cbdb5b136f6f\"}]},\"type\":\"ConnectorPlacement.EquallySpacedConnector\",\"uuid\":\"60e52eb2-18eb-41a9-88d9-70caa688cc15\"}],\"packageUris\":[\"http://schema.mathworks.com/mf0/Connector/R2020b\"],\"version\":\"1.0\"}"
      mask Display: image('E:\Hoc\do an\(final) download\test14\image\wheel.png'); % Use "Edit Image" on toolstrip to change.
  World : Subsystem
  pinion_1_RIGID : Subsystem
      settings: PortSchema="{\"entries\":[{\"content\":{\"sides\":[{\"content\":{\"connectorIds\":[\"LConn1\",\"LConn2\"]},\"type\":\"ConnectorPlacement.EquallySpacedRectSide\",\"uuid\":\"f74e51c9-4483-41be-a5a0-a0b9d89f21d7\"},{\"content\":{\"connectorIds\":[],\"side\":\"RIGHT\"},\"type\":\"ConnectorPlacement.EquallySpacedRectSide\",\"uuid\":\"cffded99-e47b-48ab-a807-0eeb52369263\"},{\"content\":{\"connectorIds\":[\"LConn3\"],\"side\":\"TOP\"},\"type\":\"ConnectorPlacement.EquallySpacedRectSide\",\"uuid\":\"87077b8b-08f2-4a0c-bdba-ac54f50e9956\"},{\"content\":{\"connectorIds\":[\"RConn1\"],\"side\":\"BOTTOM\"},\"type\":\"ConnectorPlacement.EquallySpacedRectSide\",\"uuid\":\"9d3dcba3-fa6c-4e19-8dd5-942df39ec741\"}]},\"type\":\"ConnectorPlacement.EquallySpacedConnector\",\"uuid\":\"fa2ae73f-5a1c-43be-adcd-a3eea136056e\"}],\"packageUris\":[\"http://schema.mathworks.com/mf0/Connector/R2020b\"],\"version\":\"1.0\"}"
      mask Display: image('E:\Hoc\do an\(final) download\test14\image\pinion.png'); % Use "Edit Image" on toolstrip to change.
  F : PMIOPort  Side=Left
  Steering angle left : Outport
  Steering angle right : Outport  Port=2
  wires:
  "Sensing "/2(Steering angle right (rad)) -> Steering angle right/1
  "Sensing "/1(Steering angle left (rad)) -> Steering angle left/1
  Steer angle from driver/1 -> Chassis + Rack/1(Steer angle from driver)
  "Resistance torque on left wheel "/1 -> Simulink-PS Converter1/1
  "Resistance torque on right wheel "/1 -> Simulink-PS Converter2/1
  connections:
  Revolute1/RConn1 -- Wheel Right/LConn1
  Revolute/LConn1 -- Wheel Left/RConn1
  Revolute/RConn1 -- Stability Bar/LConn1
  Chassis + Rack/LConn3 -- pinion_1_RIGID/RConn1
  Steering_wheel/LConn1 -- Rod_2_RIGID/LConn1
  Revolute1/LConn1 -- Stability Bar/RConn1
  Rack and Pinion Constraint/RConn1 -- Chassis + Rack/LConn1
  Revolute/RConn2 -- "Sensing "/LConn1
  pinion_1_RIGID/LConn1 -- F/RConn1
  Chassis + Rack/RConn1 -- Wheel Left/LConn1
  Rod_2_RIGID/RConn1 -- pinion_1_RIGID/LConn3
  Revolute1/RConn2 -- "Sensing "/LConn2
  Chassis + Rack/LConn2 -- World/LConn1 -- Transform1/LConn1
  Transform1/RConn1 -- Stability Bar/LConn2
  Chassis + Rack/RConn2 -- Wheel Right/LConn2
  Rack and Pinion Constraint/LConn1 -- pinion_1_RIGID/LConn2
  Simulink-PS Converter1/RConn1 -- Revolute/LConn2
  Simulink-PS Converter2/RConn1 -- Revolute1/LConn2

== system FinalTest_21_3/Tire Forces/Normal and Longitudinal force Area/Normal Force ==
  In1 : Inport
  A2/l : Subsystem
  Acceleration Conversion : aerolibconvert2/Acceleration Conversion  IU=m/s^2  OU=m/s^2
  Gain : Gain  Gain=1/2
  Product : Product  Inputs=3
  gravity : Constant  Value=9.81
  Fz : Outport
  wires:
  Gain/1 -> Fz/1  "Fz"
  Product/1 -> Gain/1
  gravity/1 -> Acceleration Conversion/1
  A2/l/1(Out1) -> Product/3
  In1/1 -> Product/1  "Vehicle mass"
  Acceleration Conversion/1 -> Product/2

== system FinalTest_21_3/Tire Forces/Lateral Force Area/Steering system without Tire/Chassis + Rack ==
  Steer angle from driver : Inport
  Rack Case + Chassis : Subsystem
      settings: PortSchema="{\"entries\":[{\"content\":{\"sides\":[{\"content\":{\"connectorIds\":[\"LConn1\",\"LConn2\",\"LConn3\",\"LConn4\",\"LConn5\",\"LConn6\",\"In1\"]},\"type\":\"ConnectorPlacement.EquallySpacedRectSide\",\"uuid\":\"ed584127-9069-4c16-9925-38a6e557aeb3\"},{\"content\":{\"connectorIds\":[\"RConn1\"],\"side\":\"RIGHT\"},\"type\":\"ConnectorPlacement.EquallySpacedRectSide\",\"uuid\":\"94a97d2f-d188-42ce-bea7-f0596e7c14ca\"},{\"content\":{\"connectorIds\":[\"LConn7\"],\"side\":\"TOP\"},\"type\":\"ConnectorPlacement.EquallySpacedRectSide\",\"uuid\":\"017c2ca5-4245-49bc-8ef6-d6ad1a37bd1b\"},{\"content\":{\"connectorIds\":[\"RConn2\"],\"side\":\"BOTTOM\"},\"type\":\"ConnectorPlacement.EquallySpacedRectSide\",\"uuid\":\"0bd709a1-ccd5-4aa5-ac63-3af360e493cd\"}]},\"type\":\"ConnectorPlacement.EquallySpacedConnector\",\"uuid\":\"83a19570-9384-4761-b7e7-7c808774956a\"}],\"packageUris\":[\"http://schema.mathworks.com/mf0/Connector/R2020b\"],\"version\":\"1.0\"}"
  Rack_1_RIGID : Subsystem
  Target : PMIOPort  Side=Left
  Conn3 : PMIOPort  Port=2  Side=Left
  Conn1 : PMIOPort  Port=3  Side=Left
  F2 : PMIOPort  Port=4  Side=Right
  F3 : PMIOPort  Port=5  Side=Right
  wires:
  Steer angle from driver/1 -> Rack Case + Chassis/1(Steer angle from driver)
  connections:
  Rack_1_RIGID/RConn1 -- Rack Case + Chassis/LConn2
  Rack_1_RIGID/RConn2 -- Rack Case + Chassis/LConn3
  Rack_1_RIGID/RConn4 -- Rack Case + Chassis/LConn5
  Conn3/RConn1 -- Rack Case + Chassis/LConn1
  Target/RConn1 -- Rack_1_RIGID/LConn1
  Rack Case + Chassis/LConn4 -- Rack_1_RIGID/RConn3
  Rack Case + Chassis/LConn7 -- F2/RConn1
  Rack Case + Chassis/LConn6 -- Rack_1_RIGID/RConn5
  Rack Case + Chassis/RConn2 -- F3/RConn1
  Rack Case + Chassis/RConn1 -- Conn1/RConn1

== system FinalTest_21_3/Tire Forces/Lateral Force Area/Steering system without Tire/Rod_2_RIGID ==
  ReferenceFrame : sm_lib/Frames and Transforms/Reference Frame
  Solid : sm_lib/Body Elements/File Solid  ExtGeomFileName=Rod_Default_sldprt.STEP  UnitType=FromFile  ExtGeomFileUnits=m  StepReaderType=HEX  ExportConvexHullGeometry=off  InertiaType=Custom  Mass=smiData.Solid(4).mass  MassUnits=kg  CenterOfMass=smiData.Solid(4).CoM  CenterOfMassUnits=mm  MomentsOfInertia=smiData.Solid(4).MoI  MomentsOfInertiaUnits=kg*mm^2  ProductsOfInertia=smiData.Solid(4).PoI  ProductsOfInertiaUnits=kg*mm^2  BasedOnType=DensityFromFile  Density=1000  DensityUnits=kg/m^3  DoExposeReferenceFrame=on  SerializedFrames=<Frames/>  GraphicType=FromGeometry  MarkerShape=Sphere  MarkerSize=10  GraphicVisPropType=SimpleVisualProperties  GraphicDiffuseColor=smiData.Solid(4).color  GraphicSpecularColor=[0.5 0.5 0.5 1.0]  GraphicAmbientColor=[0.15 0.15 0.15 1.0]  GraphicEmissiveColor=[0.0 0.0 0.0 1.0]  GraphicShininess=75  GraphicOpacity=smiData.Solid(4).opacity
  Transform : sm_lib/Frames and Transforms/Rigid Transform  TranslationMethod=Cartesian  TranslationStandardOffset=0  TranslationLengthUnit=mm  TranslationStandardAxis=+Z  TranslationCartesianOffset=smiData.RigidTransform(39).translation  TranslationROffset=0  TranslationROffsetUnits=m  TranslationZOffset=0  TranslationZOffsetUnits=m  TranslationThetaOffset=0  TranslationThetaOffsetUnits=deg  RotationMethod=ArbitraryAxis  RotationAngleUnits=rad  RotationStandardAxis=+Z  RotationAngle=smiData.RigidTransform(39).angle  RotationArbitraryAxis=smiData.RigidTransform(39).axis  FollAlignAxisA=+X  BaseAlignAxisA=+Y  FollAlignAxisB=+Y  BaseAlignAxisB=+Z  RotationSequenceAxes=FollowerAxes  RotationSequence=XYX  RotationSequenceAngles=[0 0 0]  RotationSequenceAnglesUnits=deg  RotationMatrix=[1 0 0; 0 1 0; 0 0 1]  Quaternion=[1 0 0 0]
  Transform1 : sm_lib/Frames and Transforms/Rigid Transform  TranslationMethod=Cartesian  TranslationStandardOffset=0  TranslationLengthUnit=mm  TranslationStandardAxis=+Z  TranslationCartesianOffset=smiData.RigidTransform(42).translation  TranslationROffset=0  TranslationROffsetUnits=m  TranslationZOffset=0  TranslationZOffsetUnits=m  TranslationThetaOffset=0  TranslationThetaOffsetUnits=deg  RotationMethod=ArbitraryAxis  RotationAngleUnits=rad  RotationStandardAxis=+Z  RotationAngle=smiData.RigidTransform(42).angle  RotationArbitraryAxis=smiData.RigidTransform(42).axis  FollAlignAxisA=+X  BaseAlignAxisA=+Y  FollAlignAxisB=+Y  BaseAlignAxisB=+Z  RotationSequenceAxes=FollowerAxes  RotationSequence=XYX  RotationSequenceAngles=[0 0 0]  RotationSequenceAnglesUnits=deg  RotationMatrix=[1 0 0; 0 1 0; 0 0 1]  Quaternion=[1 0 0 0]
  F : PMIOPort  Side=Left
  F1 : PMIOPort  Port=2  Side=Right
  connections:
  Solid/RConn1 -- ReferenceFrame/RConn1 -- Transform/LConn1 -- Transform1/LConn1
  Transform/RConn1 -- F/RConn1
  Transform1/RConn1 -- F1/RConn1

== system FinalTest_21_3/Tire Forces/Lateral Force Area/Steering system without Tire/Sensing  ==
  Add : Sum
  Add1 : Sum
  Constant1 : Constant  Value=1.57
  Constant2 : Constant  Value=1.57
  PS-Simulink Converter : nesl_utility/PS-Simulink Converter  PhysicalDomain=network_engine_domain  SubClassName=ps_output  LeftPortType=input  RightPortType=output  PseudoPeriodic=off  Frequencies=[]  VectorFormat=inherit  Unit=rad  AffineConversion=off
  PS-Simulink Converter1 : nesl_utility/PS-Simulink Converter  PhysicalDomain=network_engine_domain  SubClassName=ps_output  LeftPortType=input  RightPortType=output  PseudoPeriodic=off  Frequencies=[]  VectorFormat=inherit  Unit=rad  AffineConversion=off
  input : PMIOPort  Side=Left
  input1 : PMIOPort  Port=2  Side=Left
  Steering angle left (rad) : Outport
  Steering angle right (rad) : Outport  Port=2
  wires:
  Constant1/1 -> Add/2
  PS-Simulink Converter1/1 -> Add1/1  "Steering angle right (rad)"
  PS-Simulink Converter/1 -> Add/1  "Steering angle left (rad)"
  Constant2/1 -> Add1/2
  Add/1 -> Steering angle left (rad)/1  "Steering angle left (rad)"
  Add1/1 -> Steering angle right (rad)/1  "Steering angle right (rad)"
  connections:
  input/RConn1 -- PS-Simulink Converter/LConn1
  input1/RConn1 -- PS-Simulink Converter1/LConn1

== system FinalTest_21_3/Tire Forces/Lateral Force Area/Steering system without Tire/Stability Bar ==
  ReferenceFrame : sm_lib/Frames and Transforms/Reference Frame
  Solid : sm_lib/Body Elements/File Solid  ExtGeomFileName=lock_arm by Long_Default_sldprt.STEP  UnitType=FromFile  ExtGeomFileUnits=m  StepReaderType=HEX  ExportConvexHullGeometry=off  InertiaType=Custom  Mass=smiData.Solid(12).mass  MassUnits=kg  CenterOfMass=smiData.Solid(12).CoM  CenterOfMassUnits=mm  MomentsOfInertia=smiData.Solid(12).MoI  MomentsOfInertiaUnits=kg*mm^2  ProductsOfInertia=smiData.Solid(12).PoI  ProductsOfInertiaUnits=kg*mm^2  BasedOnType=DensityFromFile  Density=1000  DensityUnits=kg/m^3  DoExposeReferenceFrame=on  SerializedFrames=<Frames/>  GraphicType=FromGeometry  MarkerShape=Sphere  MarkerSize=10  GraphicVisPropType=SimpleVisualProperties  GraphicDiffuseColor=smiData.Solid(12).color  GraphicSpecularColor=[0.5 0.5 0.5 1.0]  GraphicAmbientColor=[0.15 0.15 0.15 1.0]  GraphicEmissiveColor=[0.0 0.0 0.0 1.0]  GraphicShininess=75  GraphicOpacity=smiData.Solid(12).opacity
  Transform : sm_lib/Frames and Transforms/Rigid Transform  TranslationMethod=Cartesian  TranslationStandardOffset=0  TranslationLengthUnit=mm  TranslationStandardAxis=+Z  TranslationCartesianOffset=smiData.RigidTransform(2).translation  TranslationROffset=0  TranslationROffsetUnits=m  TranslationZOffset=0  TranslationZOffsetUnits=m  TranslationThetaOffset=0  TranslationThetaOffsetUnits=deg  RotationMethod=ArbitraryAxis  RotationAngleUnits=rad  RotationStandardAxis=+Z  RotationAngle=smiData.RigidTransform(2).angle  RotationArbitraryAxis=smiData.RigidTransform(2).axis  FollAlignAxisA=+X  BaseAlignAxisA=+Y  FollAlignAxisB=+Y  BaseAlignAxisB=+Z  RotationSequenceAxes=FollowerAxes  RotationSequence=XYX  RotationSequenceAngles=[0 0 0]  RotationSequenceAnglesUnits=deg  RotationMatrix=[1 0 0; 0 1 0; 0 0 1]  Quaternion=[1 0 0 0]
  Transform1 : sm_lib/Frames and Transforms/Rigid Transform  TranslationMethod=Cartesian  TranslationStandardOffset=0  TranslationLengthUnit=mm  TranslationStandardAxis=+Z  TranslationCartesianOffset=smiData.RigidTransform(3).translation  TranslationROffset=0  TranslationROffsetUnits=m  TranslationZOffset=0  TranslationZOffsetUnits=m  TranslationThetaOffset=0  TranslationThetaOffsetUnits=deg  RotationMethod=ArbitraryAxis  RotationAngleUnits=rad  RotationStandardAxis=+Z  RotationAngle=smiData.RigidTransform(3).angle  RotationArbitraryAxis=smiData.RigidTransform(3).axis  FollAlignAxisA=+X  BaseAlignAxisA=+Y  FollAlignAxisB=+Y  BaseAlignAxisB=+Z  RotationSequenceAxes=FollowerAxes  RotationSequence=XYX  RotationSequenceAngles=[0 0 0]  RotationSequenceAnglesUnits=deg  RotationMatrix=[1 0 0; 0 1 0; 0 0 1]  Quaternion=[1 0 0 0]
  F : PMIOPort  Side=Left
  F2 : PMIOPort  Port=2  Side=Left
  F1 : PMIOPort  Port=3  Side=Right
  connections:
  Solid/RConn1 -- ReferenceFrame/RConn1 -- Transform/LConn1 -- Transform1/LConn1 -- F2/RConn1
  Transform/RConn1 -- F/RConn1
  Transform1/RConn1 -- F1/RConn1

== system FinalTest_21_3/Tire Forces/Lateral Force Area/Steering system without Tire/Steering_wheel ==
  ReferenceFrame : sm_lib/Frames and Transforms/Reference Frame
  Solid : sm_lib/Body Elements/File Solid  ExtGeomFileName=Steering wheel_Default_sldprt.STEP  UnitType=FromFile  ExtGeomFileUnits=m  StepReaderType=HEX  ExportConvexHullGeometry=off  InertiaType=Custom  Mass=smiData.Solid(9).mass  MassUnits=kg  CenterOfMass=smiData.Solid(9).CoM  CenterOfMassUnits=mm  MomentsOfInertia=smiData.Solid(9).MoI  MomentsOfInertiaUnits=kg*mm^2  ProductsOfInertia=smiData.Solid(9).PoI  ProductsOfInertiaUnits=kg*mm^2  BasedOnType=DensityFromFile  Density=1000  DensityUnits=kg/m^3  DoExposeReferenceFrame=on  SerializedFrames=<Frames/>  GraphicType=FromGeometry  MarkerShape=Sphere  MarkerSize=10  GraphicVisPropType=SimpleVisualProperties  GraphicDiffuseColor=smiData.Solid(9).color  GraphicSpecularColor=[0.5 0.5 0.5 1.0]  GraphicAmbientColor=[0.15 0.15 0.15 1.0]  GraphicEmissiveColor=[0.0 0.0 0.0 1.0]  GraphicShininess=75  GraphicOpacity=smiData.Solid(9).opacity
  Transform : sm_lib/Frames and Transforms/Rigid Transform  TranslationMethod=Cartesian  TranslationStandardOffset=0  TranslationLengthUnit=mm  TranslationStandardAxis=+Z  TranslationCartesianOffset=smiData.RigidTransform(40).translation  TranslationROffset=0  TranslationROffsetUnits=m  TranslationZOffset=0  TranslationZOffsetUnits=m  TranslationThetaOffset=0  TranslationThetaOffsetUnits=deg  RotationMethod=ArbitraryAxis  RotationAngleUnits=rad  RotationStandardAxis=+Z  RotationAngle=smiData.RigidTransform(40).angle  RotationArbitraryAxis=smiData.RigidTransform(40).axis  FollAlignAxisA=+X  BaseAlignAxisA=+Y  FollAlignAxisB=+Y  BaseAlignAxisB=+Z  RotationSequenceAxes=FollowerAxes  RotationSequence=XYX  RotationSequenceAngles=[0 0 0]  RotationSequenceAnglesUnits=deg  RotationMatrix=[1 0 0; 0 1 0; 0 0 1]  Quaternion=[1 0 0 0]
  F : PMIOPort  Side=Left
  connections:
  Solid/RConn1 -- ReferenceFrame/RConn1 -- Transform/LConn1
  Transform/RConn1 -- F/RConn1

== system FinalTest_21_3/Tire Forces/Lateral Force Area/Steering system without Tire/Wheel Left ==
  Innova_Crysta_Assembly_Final_1_RIGID : Subsystem
  wheelpin_by_Long_1_RIGID : Subsystem
  F2 : PMIOPort  Side=Left
  F : PMIOPort  Port=2  Side=Right
  connections:
  Innova_Crysta_Assembly_Final_1_RIGID/RConn1 -- wheelpin_by_Long_1_RIGID/LConn1
  F2/RConn1 -- wheelpin_by_Long_1_RIGID/RConn2
  F/RConn1 -- wheelpin_by_Long_1_RIGID/RConn1

== system FinalTest_21_3/Tire Forces/Lateral Force Area/Steering system without Tire/Wheel Right ==
  Innova_Crysta_Assembly_Final_2_RIGID : Subsystem
  wheelpin_by_Long_2_RIGID : Subsystem
  F : PMIOPort  Side=Left
  F2 : PMIOPort  Port=2  Side=Left
  connections:
  Innova_Crysta_Assembly_Final_2_RIGID/RConn1 -- wheelpin_by_Long_2_RIGID/RConn1
  F2/RConn1 -- wheelpin_by_Long_2_RIGID/LConn2
  F/RConn1 -- wheelpin_by_Long_2_RIGID/LConn1

== system FinalTest_21_3/Tire Forces/Lateral Force Area/Steering system without Tire/World ==
  MechanismConfiguration : sm_lib/Utilities/Mechanism Configuration  UniformGravity=Constant  GravityVector=[0 -9.80665 0]  GravityUnits=m/s^2  LinearizationDelta=0.001  JointModeTransitionNonlinearIterations=2
  Solver Configuration : nesl_utility/Solver Configuration  PhysicalDomain=network_engine_domain  SubClassName=solver  LeftPortType=input  RightPortType=generic  Tones=[]  Harmonics=[]  SimulateNoise=off  Profile=off  UseLocalSampling=off  EnableSwitchedLinearOptims=on  FrequencyDomain=off  UseCCode=off  RelTol=0.001  AbsTol=0.001  MinStep=1e-09  ToWorkspace=off  RevertToSquareIcSolve=off  NumHomotopyIterations=100  PhasorMode=off  PhasorModeNumHarmonics=1  ConsistencySolver=NEWTON_XTOL_AFTER_FTOL  IndexReductionMethod=DerivativeReplacement  DoDC=off  ResidualTolerance=1e-09  ConsistencyTolSource=GLOBAL  ConsistencyAbsTol=0.001  ConsistencyRelTol=0.001  ConsistencyTolFactor=0.001  UseLocalSolver=off  LocalSolverChoice=NE_BACKWARD_EULER_ADVANCER  ResolveIndetEquations=on  FunctionEvalNumThread=1  LocalSolverSampleTime=0.001  DoFixedCost=off  MaxNonlinIter=3  MaxModeIter=2  ComputeImpulses=off  ImpulseIterations=2  LinearAlgebra=auto  LinearAlgebraNumThread=0  EquationFormulation=NE_TIME_EF  DelaysMemoryBudget=1024  AutomaticFiltering=on  FilteringTimeConstant=0.001  PartitionStorageMethod=AS_NEEDED  PartitionMemoryBudget=1024  PartitionMethod=ROBUST
  World : sm_lib/Frames and Transforms/World Frame
  Conn1 : PMIOPort  Side=Left
  connections:
  MechanismConfiguration/RConn1 -- Conn1/RConn1 -- World/RConn1 -- Solver Configuration/RConn1
